simulink model "example3"  (R2024a)
settings: Solver=VariableStepAuto  StartTime=0.0  StopTime=10.0  RelTol=1e-3
libraries: simulink x1
settings Model: Creator=guirl  LastModifiedBy=guirl

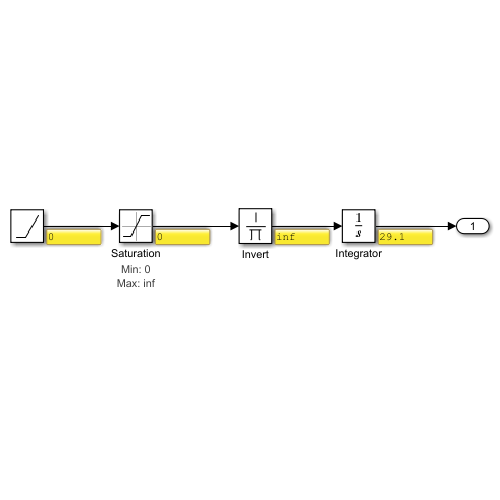
[thumbnail: Simulink's stored preview of the top-level diagram]
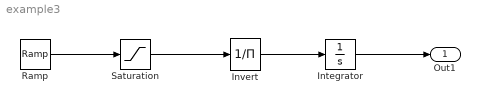
== system example3 ==
  Integrator : Integrator
  Invert : Product  Inputs=/
  Ramp : simulink/Sources/Ramp  slope=-1.123  start=0  InitialOutput=1
  Saturation : Saturate  UpperLimit=inf  LowerLimit=0
      settings: AttributesFormatString=|
      | Min: %<LowerLimit>
      | Max: %<UpperLimit>
  Out1 : Outport
  wires:
  Ramp/1 -> Saturation/1
  Integrator/1 -> Out1/1
  Saturation/1 -> Invert/1
  Invert/1 -> Integrator/1
